simulink model "RBD_sim_model"  (R2023b)
settings: Solver=ode4  StartTime=t0  StopTime=tf  FixedStep=dt  RelTol=1e-3
undefined symbols (not defined in the file): F_gravity_0, gravity, M_0, mass, p0, phi0, psi0, q0, r0, theta0, u0, v0, w0, x0, y0, z0
libraries: shared6dof x1, aerolibasang x1, dspsigops x1
settings Model: Creator=Ahmed Raamadan  LastModifiedBy=Ahmed Raamadan

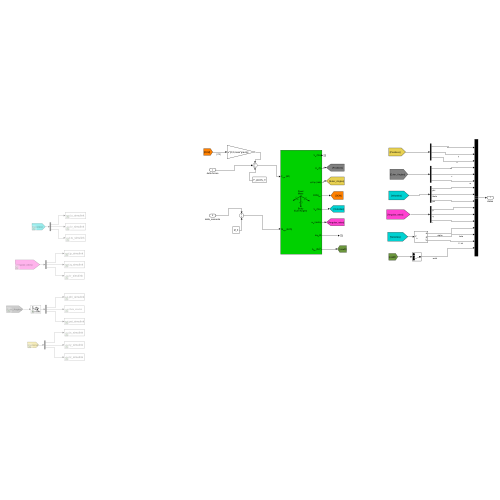
[thumbnail: Simulink's stored preview of the top-level diagram]
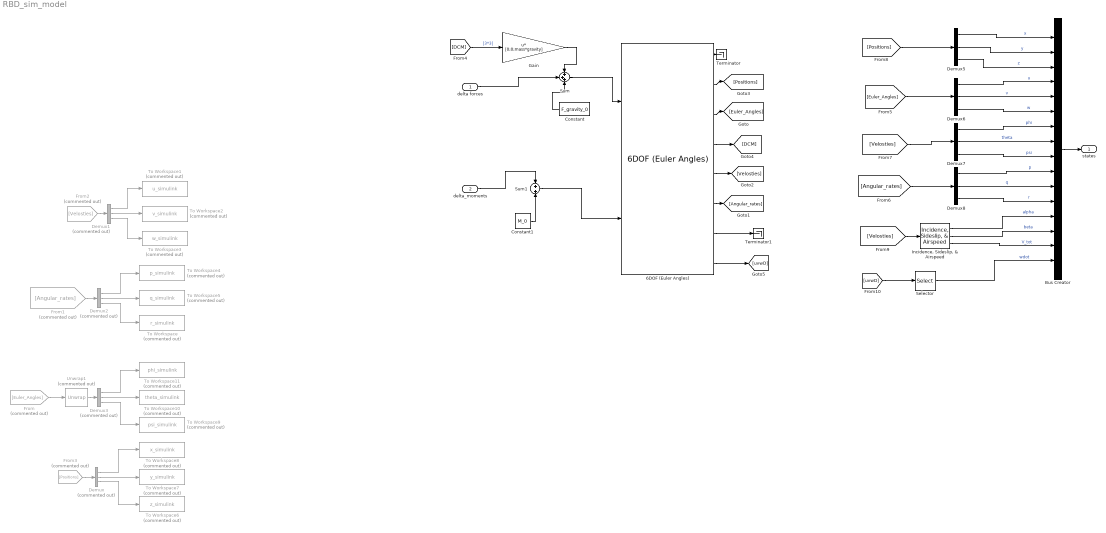
== system RBD_sim_model ==
  delta forces : Inport
  delta_moments : Inport  Port=2
  6DOF (Euler Angles) : shared6dof/6DOF (Euler Angles)  units=English (Velocity in ft/s)  mtype=Fixed  rep=Euler Angles  xme_0=[x0 y0 z0]  Vm_0=[u0 v0 w0]  eul_0=[phi0 theta0 psi0]  pm_0=[p0 q0 r0]  mass_0=mass  mass_e=0.5  mass_f=2.0  inertia=Inertia  inertia_e=eye(3)  inertia_f=2*eye(3)  k_quat=1.0  vre_flag=on  abi_flag=off  aMode=0  xme_statename=''  Vm_statename=''  eul_statename=''  quat_statename=''  pm_statename=''  mass_statename=''
  Bus Creator : BusCreator  Inputs=16
  Constant : Constant  Value=F_gravity_0
  Constant1 : Constant  Value=M_0
  Demux{,1..3} (4 alike) : Demux  Commented=on  Outputs=3
  Demux{5..8} (4 alike) : Demux  Outputs=3
  From : From  Commented=on  GotoTag=Euler_Angles
  From1 : From  Commented=on  GotoTag=Angular_rates
  From2 : From  Commented=on  GotoTag=Velosties
  From3 : From  Commented=on  GotoTag=Positions
  Gain : Gain  Gain=[0;0;mass*gravity]  Multiplication=Matrix(u*K)
  "Incidence, Sideslip, & Airspeed" : aerolibasang/Incidence, Sideslip, & Airspeed
  Selector : Selector  InputPortWidth=3  IndexOptions=Index vector (dialog)  Indices=[3]  OutputSizes=1  RuntimeRangeChecks=on
  Sum : Sum  Inputs=+++
  Sum1 : Sum
  Terminator : Terminator
  Terminator1 : Terminator
  To Workspace : ToWorkspace  Commented=on  VariableName=r_simulink  SaveFormat=Timeseries  SampleTime=-1
  To Workspace1 : ToWorkspace  Commented=on  VariableName=u_simulink  SaveFormat=Timeseries  SampleTime=-1
  To Workspace10 : ToWorkspace  Commented=on  VariableName=theta_simulink  SaveFormat=Timeseries  SampleTime=-1
  To Workspace11 : ToWorkspace  Commented=on  VariableName=phi_simulink  SaveFormat=Timeseries  SampleTime=-1
  To Workspace2 : ToWorkspace  Commented=on  VariableName=v_simulink  SaveFormat=Timeseries  SampleTime=-1
  To Workspace3 : ToWorkspace  Commented=on  VariableName=w_simulink  SaveFormat=Timeseries  SampleTime=-1
  To Workspace4 : ToWorkspace  Commented=on  VariableName=p_simulink  SaveFormat=Timeseries  SampleTime=-1
  To Workspace5 : ToWorkspace  Commented=on  VariableName=q_simulink  SaveFormat=Timeseries  SampleTime=-1
  To Workspace6 : ToWorkspace  Commented=on  VariableName=z_simulink  SaveFormat=Timeseries  SampleTime=-1
  To Workspace7 : ToWorkspace  Commented=on  VariableName=y_simulink  SaveFormat=Timeseries  SampleTime=-1
  To Workspace8 : ToWorkspace  Commented=on  VariableName=x_simulink  SaveFormat=Timeseries  SampleTime=-1
  To Workspace9 : ToWorkspace  Commented=on  VariableName=psi_simulink  SaveFormat=Timeseries  SampleTime=-1
  Unwrap1 : dspsigops/Unwrap  Commented=on  tol=pi  running=off
  states : Outport
  wires:
  Demux/1 -> To Workspace8/1
  Demux/2 -> To Workspace7/1
  Demux/3 -> To Workspace6/1
  Demux1/1 -> To Workspace1/1
  Demux1/3 -> To Workspace3/1
  Demux1/2 -> To Workspace2/1
  Demux2/1 -> To Workspace4/1
  Demux2/2 -> To Workspace5/1
  Demux2/3 -> To Workspace/1
  Demux3/3 -> To Workspace9/1
  Demux3/2 -> To Workspace10/1
  Demux3/1 -> To Workspace11/1
  6DOF (Euler Angles)/6 -> [Angular_rates]
  6DOF (Euler Angles)/3 -> [Euler_Angles]
  From/1 -> Unwrap1/1
  Unwrap1/1 -> Demux3/1
  From1/1 -> Demux2/1
  6DOF (Euler Angles)/5 -> [Velosties]
  From2/1 -> Demux1/1
  6DOF (Euler Angles)/2 -> [Positions]
  From3/1 -> Demux/1
  6DOF (Euler Angles)/1 -> Terminator/1
  6DOF (Euler Angles)/4 -> [DCM]
  [DCM] -> Gain/1  "[3*3]"
  Gain/1 -> Sum/1
  6DOF (Euler Angles)/8 -> [uvwD]
  6DOF (Euler Angles)/7 -> Terminator1/1
  [Velosties] -> "Incidence, Sideslip, & Airspeed"/1
  [uvwD] -> Selector/1
  [Positions] -> Demux5/1
  Demux5/1 -> Bus Creator/1  "x"
  Demux5/2 -> Bus Creator/2  "y"
  Demux5/3 -> Bus Creator/3  "z"
  Demux6/1 -> Bus Creator/4  "u"
  Demux6/3 -> Bus Creator/6  "w"
  [Euler_Angles] -> Demux6/1
  Demux6/2 -> Bus Creator/5  "v"
  [Velosties] -> Demux7/1
  Demux7/1 -> Bus Creator/7  "phi"
  Demux7/2 -> Bus Creator/8  "theta"
  Demux7/3 -> Bus Creator/9  "psi"
  [Angular_rates] -> Demux8/1
  Demux8/1 -> Bus Creator/10  "p"
  Demux8/2 -> Bus Creator/11  "q"
  Demux8/3 -> Bus Creator/12  "r"
  "Incidence, Sideslip, & Airspeed"/1 -> Bus Creator/13  "alpha"
  "Incidence, Sideslip, & Airspeed"/2 -> Bus Creator/14  "beta"
  "Incidence, Sideslip, & Airspeed"/3 -> Bus Creator/15  "V_tot"
  Selector/1 -> Bus Creator/16  "wdot"
  delta forces/1 -> Sum/2
  delta_moments/1 -> Sum1/1
  Constant/1 -> Sum/3
  Sum/1 -> 6DOF (Euler Angles)/1
  Constant1/1 -> Sum1/2
  Sum1/1 -> 6DOF (Euler Angles)/2
  Bus Creator/1 -> states/1
